simulink model "AA_Assemblage"  (R2020b)
settings: Solver=FixedStepAuto  StartTime=0.0  StopTime=inf  FixedStep=0.001  RelTol=1e-3
values from neighbouring files (symbols this model uses):
  smiData =     [A_robot_move.mat]
undefined symbols (not defined in the file or in its folder): Levenberg, Marquardt, W, X, Y, Z
libraries: sm_lib x1154, nesl_utility x40, robotlib x9, robotmaniplib x4, robotcorelib x2, simulink x1
(part 5 of 19)

== system AA_Assemblage/Robot_consigne/Poignet_1/SKF_7202_1_RIGID ==
  ReferenceFrame : sm_lib/Frames and Transforms/Reference Frame
  Solid : sm_lib/Body Elements/File Solid  ExtGeomFileName=SKF 7202.step  UnitType=FromFile  ExtGeomFileUnits=m  StepReaderType=HEX  ExportConvexHullGeometry=off  InertiaType=Custom  Mass=smiData.Solid(18).mass  MassUnits=kg  CenterOfMass=smiData.Solid(18).CoM  CenterOfMassUnits=mm  MomentsOfInertia=smiData.Solid(18).MoI  MomentsOfInertiaUnits=kg*mm^2  ProductsOfInertia=smiData.Solid(18).PoI  ProductsOfInertiaUnits=kg*mm^2  BasedOnType=DensityFromFile  Density=1000  DensityUnits=kg/m^3  DoExposeReferenceFrame=on  SerializedFrames=<Frames/>  GraphicType=FromGeometry  MarkerShape=Sphere  MarkerSize=10  GraphicVisPropType=SimpleVisualProperties  GraphicDiffuseColor=smiData.Solid(18).color  GraphicSpecularColor=[0.5 0.5 0.5 1.0]  GraphicAmbientColor=[0.15 0.15 0.15 1.0]  GraphicEmissiveColor=[0.0 0.0 0.0 1.0]  GraphicShininess=75  GraphicOpacity=smiData.Solid(18).opacity
  Transform : sm_lib/Frames and Transforms/Rigid Transform  TranslationMethod=Cartesian  TranslationStandardOffset=0  TranslationLengthUnit=mm  TranslationStandardAxis=+Z  TranslationCartesianOffset=smiData.RigidTransform(68).translation  TranslationROffset=0  TranslationROffsetUnits=m  TranslationZOffset=0  TranslationZOffsetUnits=m  TranslationThetaOffset=0  TranslationThetaOffsetUnits=deg  RotationMethod=ArbitraryAxis  RotationAngleUnits=rad  RotationStandardAxis=+Z  RotationAngle=smiData.RigidTransform(68).angle  RotationArbitraryAxis=smiData.RigidTransform(68).axis  FollAlignAxisA=+X  BaseAlignAxisA=+Y  FollAlignAxisB=+Y  BaseAlignAxisB=+Z  RotationSequenceAxes=FollowerAxes  RotationSequence=XYX  RotationSequenceAngles=[0 0 0]  RotationSequenceAnglesUnits=deg  RotationMatrix=[1 0 0; 0 1 0; 0 0 1]
  F : PMIOPort  Side=Left
  connections:
  ReferenceFrame/RConn1 -- Solid/RConn1 -- Transform/LConn1
  Transform/RConn1 -- F/RConn1

== system AA_Assemblage/Robot_consigne/Poignet_1/SKF_7202_2_RIGID ==
  ReferenceFrame : sm_lib/Frames and Transforms/Reference Frame
  Solid : sm_lib/Body Elements/File Solid  ExtGeomFileName=SKF 7202.step  UnitType=FromFile  ExtGeomFileUnits=m  StepReaderType=HEX  ExportConvexHullGeometry=off  InertiaType=Custom  Mass=smiData.Solid(18).mass  MassUnits=kg  CenterOfMass=smiData.Solid(18).CoM  CenterOfMassUnits=mm  MomentsOfInertia=smiData.Solid(18).MoI  MomentsOfInertiaUnits=kg*mm^2  ProductsOfInertia=smiData.Solid(18).PoI  ProductsOfInertiaUnits=kg*mm^2  BasedOnType=DensityFromFile  Density=1000  DensityUnits=kg/m^3  DoExposeReferenceFrame=on  SerializedFrames=<Frames/>  GraphicType=FromGeometry  MarkerShape=Sphere  MarkerSize=10  GraphicVisPropType=SimpleVisualProperties  GraphicDiffuseColor=smiData.Solid(18).color  GraphicSpecularColor=[0.5 0.5 0.5 1.0]  GraphicAmbientColor=[0.15 0.15 0.15 1.0]  GraphicEmissiveColor=[0.0 0.0 0.0 1.0]  GraphicShininess=75  GraphicOpacity=smiData.Solid(18).opacity
  Transform : sm_lib/Frames and Transforms/Rigid Transform  TranslationMethod=Cartesian  TranslationStandardOffset=0  TranslationLengthUnit=mm  TranslationStandardAxis=+Z  TranslationCartesianOffset=smiData.RigidTransform(78).translation  TranslationROffset=0  TranslationROffsetUnits=m  TranslationZOffset=0  TranslationZOffsetUnits=m  TranslationThetaOffset=0  TranslationThetaOffsetUnits=deg  RotationMethod=ArbitraryAxis  RotationAngleUnits=rad  RotationStandardAxis=+Z  RotationAngle=smiData.RigidTransform(78).angle  RotationArbitraryAxis=smiData.RigidTransform(78).axis  FollAlignAxisA=+X  BaseAlignAxisA=+Y  FollAlignAxisB=+Y  BaseAlignAxisB=+Z  RotationSequenceAxes=FollowerAxes  RotationSequence=XYX  RotationSequenceAngles=[0 0 0]  RotationSequenceAnglesUnits=deg  RotationMatrix=[1 0 0; 0 1 0; 0 0 1]
  Transform1 : sm_lib/Frames and Transforms/Rigid Transform  TranslationMethod=Cartesian  TranslationStandardOffset=0  TranslationLengthUnit=mm  TranslationStandardAxis=+Z  TranslationCartesianOffset=smiData.RigidTransform(97).translation  TranslationROffset=0  TranslationROffsetUnits=m  TranslationZOffset=0  TranslationZOffsetUnits=m  TranslationThetaOffset=0  TranslationThetaOffsetUnits=deg  RotationMethod=ArbitraryAxis  RotationAngleUnits=rad  RotationStandardAxis=+Z  RotationAngle=smiData.RigidTransform(97).angle  RotationArbitraryAxis=smiData.RigidTransform(97).axis  FollAlignAxisA=+X  BaseAlignAxisA=+Y  FollAlignAxisB=+Y  BaseAlignAxisB=+Z  RotationSequenceAxes=FollowerAxes  RotationSequence=XYX  RotationSequenceAngles=[0 0 0]  RotationSequenceAnglesUnits=deg  RotationMatrix=[1 0 0; 0 1 0; 0 0 1]
  F : PMIOPort  Side=Left
  F1 : PMIOPort  Port=2  Side=Left
  connections:
  ReferenceFrame/RConn1 -- Solid/RConn1 -- Transform/LConn1 -- Transform1/LConn1
  Transform/RConn1 -- F/RConn1
  Transform1/RConn1 -- F1/RConn1

== system AA_Assemblage/Robot_consigne/Poignet_1/Support_Rou_dente_coude_et_poignet_1_RIGID ==
  ReferenceFrame : sm_lib/Frames and Transforms/Reference Frame
  Solid : sm_lib/Body Elements/File Solid  ExtGeomFileName=Support Roué dentée coude et poignet.step  UnitType=FromFile  ExtGeomFileUnits=m  StepReaderType=HEX  ExportConvexHullGeometry=off  InertiaType=Custom  Mass=smiData.Solid(17).mass  MassUnits=kg  CenterOfMass=smiData.Solid(17).CoM  CenterOfMassUnits=mm  MomentsOfInertia=smiData.Solid(17).MoI  MomentsOfInertiaUnits=kg*mm^2  ProductsOfInertia=smiData.Solid(17).PoI  ProductsOfInertiaUnits=kg*mm^2  BasedOnType=DensityFromFile  Density=1000  DensityUnits=kg/m^3  DoExposeReferenceFrame=on  SerializedFrames=<Frames/>  GraphicType=FromGeometry  MarkerShape=Sphere  MarkerSize=10  GraphicVisPropType=SimpleVisualProperties  GraphicDiffuseColor=smiData.Solid(17).color  GraphicSpecularColor=[0.5 0.5 0.5 1.0]  GraphicAmbientColor=[0.15 0.15 0.15 1.0]  GraphicEmissiveColor=[0.0 0.0 0.0 1.0]  GraphicShininess=75  GraphicOpacity=smiData.Solid(17).opacity
  Transform : sm_lib/Frames and Transforms/Rigid Transform  TranslationMethod=Cartesian  TranslationStandardOffset=0  TranslationLengthUnit=mm  TranslationStandardAxis=+Z  TranslationCartesianOffset=smiData.RigidTransform(80).translation  TranslationROffset=0  TranslationROffsetUnits=m  TranslationZOffset=0  TranslationZOffsetUnits=m  TranslationThetaOffset=0  TranslationThetaOffsetUnits=deg  RotationMethod=ArbitraryAxis  RotationAngleUnits=rad  RotationStandardAxis=+Z  RotationAngle=smiData.RigidTransform(80).angle  RotationArbitraryAxis=smiData.RigidTransform(80).axis  FollAlignAxisA=+X  BaseAlignAxisA=+Y  FollAlignAxisB=+Y  BaseAlignAxisB=+Z  RotationSequenceAxes=FollowerAxes  RotationSequence=XYX  RotationSequenceAngles=[0 0 0]  RotationSequenceAnglesUnits=deg  RotationMatrix=[1 0 0; 0 1 0; 0 0 1]
  F : PMIOPort  Side=Left
  connections:
  ReferenceFrame/RConn1 -- Solid/RConn1 -- Transform/LConn1
  Transform/RConn1 -- F/RConn1

== system AA_Assemblage/Robot_consigne/Poignet_1/XL430_1_RIGID ==
  ReferenceFrame : sm_lib/Frames and Transforms/Reference Frame
  Solid : sm_lib/Body Elements/File Solid  ExtGeomFileName=XL430.step  UnitType=FromFile  ExtGeomFileUnits=m  StepReaderType=HEX  ExportConvexHullGeometry=off  InertiaType=Custom  Mass=smiData.Solid(22).mass  MassUnits=kg  CenterOfMass=smiData.Solid(22).CoM  CenterOfMassUnits=mm  MomentsOfInertia=smiData.Solid(22).MoI  MomentsOfInertiaUnits=kg*mm^2  ProductsOfInertia=smiData.Solid(22).PoI  ProductsOfInertiaUnits=kg*mm^2  BasedOnType=DensityFromFile  Density=1000  DensityUnits=kg/m^3  DoExposeReferenceFrame=on  SerializedFrames=<Frames/>  GraphicType=FromGeometry  MarkerShape=Sphere  MarkerSize=10  GraphicVisPropType=SimpleVisualProperties  GraphicDiffuseColor=smiData.Solid(22).color  GraphicSpecularColor=[0.5 0.5 0.5 1.0]  GraphicAmbientColor=[0.15 0.15 0.15 1.0]  GraphicEmissiveColor=[0.0 0.0 0.0 1.0]  GraphicShininess=75  GraphicOpacity=smiData.Solid(22).opacity
  Transform : sm_lib/Frames and Transforms/Rigid Transform  TranslationMethod=Cartesian  TranslationStandardOffset=0  TranslationLengthUnit=mm  TranslationStandardAxis=+Z  TranslationCartesianOffset=smiData.RigidTransform(76).translation  TranslationROffset=0  TranslationROffsetUnits=m  TranslationZOffset=0  TranslationZOffsetUnits=m  TranslationThetaOffset=0  TranslationThetaOffsetUnits=deg  RotationMethod=ArbitraryAxis  RotationAngleUnits=rad  RotationStandardAxis=+Z  RotationAngle=smiData.RigidTransform(76).angle  RotationArbitraryAxis=smiData.RigidTransform(76).axis  FollAlignAxisA=+X  BaseAlignAxisA=+Y  FollAlignAxisB=+Y  BaseAlignAxisB=+Z  RotationSequenceAxes=FollowerAxes  RotationSequence=XYX  RotationSequenceAngles=[0 0 0]  RotationSequenceAnglesUnits=deg  RotationMatrix=[1 0 0; 0 1 0; 0 0 1]
  Transform1 : sm_lib/Frames and Transforms/Rigid Transform  TranslationMethod=Cartesian  TranslationStandardOffset=0  TranslationLengthUnit=mm  TranslationStandardAxis=+Z  TranslationCartesianOffset=smiData.RigidTransform(79).translation  TranslationROffset=0  TranslationROffsetUnits=m  TranslationZOffset=0  TranslationZOffsetUnits=m  TranslationThetaOffset=0  TranslationThetaOffsetUnits=deg  RotationMethod=ArbitraryAxis  RotationAngleUnits=rad  RotationStandardAxis=+Z  RotationAngle=smiData.RigidTransform(79).angle  RotationArbitraryAxis=smiData.RigidTransform(79).axis  FollAlignAxisA=+X  BaseAlignAxisA=+Y  FollAlignAxisB=+Y  BaseAlignAxisB=+Z  RotationSequenceAxes=FollowerAxes  RotationSequence=XYX  RotationSequenceAngles=[0 0 0]  RotationSequenceAnglesUnits=deg  RotationMatrix=[1 0 0; 0 1 0; 0 0 1]
  F1 : PMIOPort  Side=Left
  F : PMIOPort  Port=2  Side=Left
  connections:
  ReferenceFrame/RConn1 -- Solid/RConn1 -- Transform/LConn1 -- Transform1/LConn1
  Transform/RConn1 -- F/RConn1
  Transform1/RConn1 -- F1/RConn1

== system AA_Assemblage/Subsystem1/Robot_verif/Base_1 ==
  Base_Complment_1_RIGID : Subsystem
  Couvercle_Base_1_RIGID : Subsystem
  Paroi_2_Base_1_RIGID : Subsystem
  Paroi_3_Base_1_RIGID : Subsystem
  Paroi_4_Base_1_RIGID : Subsystem
  Petite_Roue_dente_Bassin_1_RIGID : Subsystem
  ReferenceFrame : sm_lib/Frames and Transforms/Reference Frame
  ReferenceFrame1 : sm_lib/Frames and Transforms/Reference Frame
  SKF_7208_1_RIGID : Subsystem
  SKF_7208_2_RIGID : Subsystem
  Sol_Base_1_RIGID : Subsystem
  Support_Rou_dente_Base_1_RIGID : Subsystem
  Transform : sm_lib/Frames and Transforms/Rigid Transform  TranslationMethod=Cartesian  TranslationStandardOffset=0  TranslationLengthUnit=mm  TranslationStandardAxis=+Z  TranslationCartesianOffset=smiData.RigidTransform(103).translation  TranslationROffset=0  TranslationROffsetUnits=m  TranslationZOffset=0  TranslationZOffsetUnits=m  TranslationThetaOffset=0  TranslationThetaOffsetUnits=deg  RotationMethod=ArbitraryAxis  RotationAngleUnits=rad  RotationStandardAxis=+Z  RotationAngle=smiData.RigidTransform(103).angle  RotationArbitraryAxis=smiData.RigidTransform(103).axis  FollAlignAxisA=+X  BaseAlignAxisA=+Y  FollAlignAxisB=+Y  BaseAlignAxisB=+Z  RotationSequenceAxes=FollowerAxes  RotationSequence=XYX  RotationSequenceAngles=[0 0 0]  RotationSequenceAnglesUnits=deg  RotationMatrix=[1 0 0; 0 1 0; 0 0 1]
  Transform1 : sm_lib/Frames and Transforms/Rigid Transform  TranslationMethod=Cartesian  TranslationStandardOffset=0  TranslationLengthUnit=mm  TranslationStandardAxis=+Z  TranslationCartesianOffset=smiData.RigidTransform(106).translation  TranslationROffset=0  TranslationROffsetUnits=m  TranslationZOffset=0  TranslationZOffsetUnits=m  TranslationThetaOffset=0  TranslationThetaOffsetUnits=deg  RotationMethod=ArbitraryAxis  RotationAngleUnits=rad  RotationStandardAxis=+Z  RotationAngle=smiData.RigidTransform(106).angle  RotationArbitraryAxis=smiData.RigidTransform(106).axis  FollAlignAxisA=+X  BaseAlignAxisA=+Y  FollAlignAxisB=+Y  BaseAlignAxisB=+Z  RotationSequenceAxes=FollowerAxes  RotationSequence=XYX  RotationSequenceAngles=[0 0 0]  RotationSequenceAnglesUnits=deg  RotationMatrix=[1 0 0; 0 1 0; 0 0 1]
  XL430_1_RIGID : Subsystem
  F : PMIOPort  Side=Right
  F3 : PMIOPort  Port=2  Side=Left
  connections:
  Paroi_4_Base_1_RIGID/LConn1 -- Sol_Base_1_RIGID/LConn2 -- Paroi_2_Base_1_RIGID/LConn1 -- Paroi_3_Base_1_RIGID/LConn1
  Support_Rou_dente_Base_1_RIGID/LConn2 -- XL430_1_RIGID/LConn1
  ReferenceFrame/RConn1 -- Transform/LConn1
  Couvercle_Base_1_RIGID/LConn1 -- XL430_1_RIGID/LConn2
  Base_Complment_1_RIGID/LConn3 -- Sol_Base_1_RIGID/LConn1
  Petite_Roue_dente_Bassin_1_RIGID/LConn1 -- Support_Rou_dente_Base_1_RIGID/LConn1
  Base_Complment_1_RIGID/LConn1 -- Couvercle_Base_1_RIGID/LConn3
  Base_Complment_1_RIGID/LConn2 -- SKF_7208_1_RIGID/LConn2
  Base_Complment_1_RIGID/LConn4 -- SKF_7208_2_RIGID/LConn1
  SKF_7208_1_RIGID/LConn1 -- F/RConn1
  Couvercle_Base_1_RIGID/LConn2 -- Transform/RConn1
  F3/RConn1 -- Transform1/LConn1 -- ReferenceFrame1/RConn1
  Transform1/RConn1 -- Sol_Base_1_RIGID/LConn3

== system AA_Assemblage/Subsystem1/Robot_verif/Coude_1 ==
  Adaptateur_Arbre_01_1_RIGID : Subsystem
  Arbre_1_1_RIGID : Subsystem
  Bras_1_droite_1_RIGID : Subsystem
  Bras_1_gauche_1_RIGID : Subsystem
  Grande_Roue_dente_paule_1_RIGID : Subsystem
  Petite_Roue_dente_Coude_1_RIGID : Subsystem
  ReferenceFrame : sm_lib/Frames and Transforms/Reference Frame
  SKF_7202_1_RIGID : Subsystem
  SKF_7202_2_RIGID : Subsystem
  Support_Rou_dente_coude_et_poignet_1_RIGID : Subsystem
  XL430_1_RIGID : Subsystem
  F1 : PMIOPort  Side=Left
  F : PMIOPort  Port=2  Side=Right
  connections:
  Bras_1_droite_1_RIGID/LConn2 -- SKF_7202_1_RIGID/LConn2
  Bras_1_droite_1_RIGID/LConn1 -- XL430_1_RIGID/LConn2
  Adaptateur_Arbre_01_1_RIGID/LConn2 -- F1/RConn1
  Arbre_1_1_RIGID/LConn2 -- Bras_1_droite_1_RIGID/LConn3
  Support_Rou_dente_coude_et_poignet_1_RIGID/LConn2 -- XL430_1_RIGID/LConn1
  Adaptateur_Arbre_01_1_RIGID/LConn3 -- Grande_Roue_dente_paule_1_RIGID/LConn1
  Arbre_1_1_RIGID/LConn1 -- Bras_1_gauche_1_RIGID/LConn2
  Adaptateur_Arbre_01_1_RIGID/LConn1 -- Arbre_1_1_RIGID/LConn3
  Bras_1_gauche_1_RIGID/LConn1 -- SKF_7202_2_RIGID/LConn1
  Petite_Roue_dente_Coude_1_RIGID/LConn1 -- Support_Rou_dente_coude_et_poignet_1_RIGID/LConn1
  SKF_7202_1_RIGID/LConn1 -- F/RConn1

== system AA_Assemblage/Subsystem1/Robot_verif/Epaule_1 ==
  Bras_01_droite_3_RIGID : Subsystem
  Bras_01_gauche_4_RIGID : Subsystem
  Mt_1_RIGID : Subsystem
  Part_2_1_RIGID : Subsystem
  Petite_Roue_dente_paule_1_RIGID : Subsystem
  Plateau_complmentaire_du_mt_2_RIGID : Subsystem
  ReferenceFrame : sm_lib/Frames and Transforms/Reference Frame
  SKF_7202_1_RIGID : Subsystem
  SKF_7202_2_RIGID : Subsystem
  XL430_1_RIGID : Subsystem
  F1 : PMIOPort  Side=Left
  F : PMIOPort  Port=2  Side=Right
  connections:
  Petite_Roue_dente_paule_1_RIGID/LConn1 -- XL430_1_RIGID/LConn1
  Mt_1_RIGID/LConn5 -- Part_2_1_RIGID/LConn1
  Bras_01_gauche_4_RIGID/LConn3 -- Mt_1_RIGID/LConn2
  Mt_1_RIGID/LConn4 -- Plateau_complmentaire_du_mt_2_RIGID/LConn1
  Bras_01_droite_3_RIGID/LConn2 -- Mt_1_RIGID/LConn1
  Bras_01_gauche_4_RIGID/LConn1 -- XL430_1_RIGID/LConn2
  Bras_01_gauche_4_RIGID/LConn2 -- SKF_7202_2_RIGID/LConn1
  Bras_01_droite_3_RIGID/LConn1 -- SKF_7202_1_RIGID/LConn2
  SKF_7202_1_RIGID/LConn1 -- F/RConn1
  Mt_1_RIGID/LConn3 -- F1/RConn1

== system AA_Assemblage/Subsystem1/Robot_verif/Main_1 ==
  Arbre_Poignet_1_RIGID : Subsystem
  Main_assemble_1 : Subsystem
  Poignet_1_RIGID : Subsystem
  engrenage_sortie_1_RIGID : Subsystem
  F : PMIOPort  Side=Left
  F1 : PMIOPort  Port=2  Side=Right
  connections:
  Arbre_Poignet_1_RIGID/LConn3 -- engrenage_sortie_1_RIGID/LConn1
  Main_assemble_1/LConn1 -- Poignet_1_RIGID/LConn1
  Arbre_Poignet_1_RIGID/LConn1 -- Poignet_1_RIGID/LConn2
  Arbre_Poignet_1_RIGID/LConn2 -- F/RConn1
  F1/RConn1 -- Main_assemble_1/RConn1

== system AA_Assemblage/Subsystem1/Robot_verif/Poignet_1 ==
  Bras1_1_RIGID : Subsystem
  Grande_Roue_dente_Coude_1_RIGID : Subsystem
  Part_1_1_RIGID : Subsystem
  Part_2_1_RIGID : Subsystem
  ReferenceFrame : sm_lib/Frames and Transforms/Reference Frame
  SKF_7202_1_RIGID : Subsystem
  SKF_7202_2_RIGID : Subsystem
  Support_Rou_dente_coude_et_poignet_1_RIGID : Subsystem
  XL430_1_RIGID : Subsystem
  F : PMIOPort  Side=Left
  F1 : PMIOPort  Port=2  Side=Right
  connections:
  Bras1_1_RIGID/LConn3 -- SKF_7202_1_RIGID/LConn1
  Bras1_1_RIGID/LConn2 -- Part_1_1_RIGID/LConn3
  Part_1_1_RIGID/LConn4 -- Part_2_1_RIGID/LConn1
  Grande_Roue_dente_Coude_1_RIGID/LConn1 -- Part_1_1_RIGID/LConn1
  Bras1_1_RIGID/LConn1 -- XL430_1_RIGID/LConn2
  Part_2_1_RIGID/LConn2 -- SKF_7202_2_RIGID/LConn1
  Support_Rou_dente_coude_et_poignet_1_RIGID/LConn1 -- XL430_1_RIGID/LConn1
  Part_1_1_RIGID/LConn2 -- F/RConn1
  SKF_7202_2_RIGID/LConn2 -- F1/RConn1

== system AA_Assemblage/Subsystem2/Robot_verif/Base_1 ==
  Base_Complment_1_RIGID : Subsystem
  Couvercle_Base_1_RIGID : Subsystem
  Paroi_2_Base_1_RIGID : Subsystem
  Paroi_3_Base_1_RIGID : Subsystem
  Paroi_4_Base_1_RIGID : Subsystem
  Petite_Roue_dente_Bassin_1_RIGID : Subsystem
  ReferenceFrame : sm_lib/Frames and Transforms/Reference Frame
  ReferenceFrame1 : sm_lib/Frames and Transforms/Reference Frame
  SKF_7208_1_RIGID : Subsystem
  SKF_7208_2_RIGID : Subsystem
  Sol_Base_1_RIGID : Subsystem
  Support_Rou_dente_Base_1_RIGID : Subsystem
  Transform : sm_lib/Frames and Transforms/Rigid Transform  TranslationMethod=Cartesian  TranslationStandardOffset=0  TranslationLengthUnit=mm  TranslationStandardAxis=+Z  TranslationCartesianOffset=smiData.RigidTransform(103).translation  TranslationROffset=0  TranslationROffsetUnits=m  TranslationZOffset=0  TranslationZOffsetUnits=m  TranslationThetaOffset=0  TranslationThetaOffsetUnits=deg  RotationMethod=ArbitraryAxis  RotationAngleUnits=rad  RotationStandardAxis=+Z  RotationAngle=smiData.RigidTransform(103).angle  RotationArbitraryAxis=smiData.RigidTransform(103).axis  FollAlignAxisA=+X  BaseAlignAxisA=+Y  FollAlignAxisB=+Y  BaseAlignAxisB=+Z  RotationSequenceAxes=FollowerAxes  RotationSequence=XYX  RotationSequenceAngles=[0 0 0]  RotationSequenceAnglesUnits=deg  RotationMatrix=[1 0 0; 0 1 0; 0 0 1]
  Transform1 : sm_lib/Frames and Transforms/Rigid Transform  TranslationMethod=Cartesian  TranslationStandardOffset=0  TranslationLengthUnit=mm  TranslationStandardAxis=+Z  TranslationCartesianOffset=smiData.RigidTransform(106).translation  TranslationROffset=0  TranslationROffsetUnits=m  TranslationZOffset=0  TranslationZOffsetUnits=m  TranslationThetaOffset=0  TranslationThetaOffsetUnits=deg  RotationMethod=ArbitraryAxis  RotationAngleUnits=rad  RotationStandardAxis=+Z  RotationAngle=smiData.RigidTransform(106).angle  RotationArbitraryAxis=smiData.RigidTransform(106).axis  FollAlignAxisA=+X  BaseAlignAxisA=+Y  FollAlignAxisB=+Y  BaseAlignAxisB=+Z  RotationSequenceAxes=FollowerAxes  RotationSequence=XYX  RotationSequenceAngles=[0 0 0]  RotationSequenceAnglesUnits=deg  RotationMatrix=[1 0 0; 0 1 0; 0 0 1]
  XL430_1_RIGID : Subsystem
  F : PMIOPort  Side=Right
  F3 : PMIOPort  Port=2  Side=Left
  connections:
  Paroi_3_Base_1_RIGID/LConn1 -- Paroi_4_Base_1_RIGID/LConn1 -- Sol_Base_1_RIGID/LConn2 -- Paroi_2_Base_1_RIGID/LConn1
  Support_Rou_dente_Base_1_RIGID/LConn2 -- XL430_1_RIGID/LConn1
  ReferenceFrame/RConn1 -- Transform/LConn1
  Couvercle_Base_1_RIGID/LConn1 -- XL430_1_RIGID/LConn2
  Base_Complment_1_RIGID/LConn3 -- Sol_Base_1_RIGID/LConn1
  Petite_Roue_dente_Bassin_1_RIGID/LConn1 -- Support_Rou_dente_Base_1_RIGID/LConn1
  Base_Complment_1_RIGID/LConn1 -- Couvercle_Base_1_RIGID/LConn3
  Base_Complment_1_RIGID/LConn2 -- SKF_7208_1_RIGID/LConn2
  Base_Complment_1_RIGID/LConn4 -- SKF_7208_2_RIGID/LConn1
  SKF_7208_1_RIGID/LConn1 -- F/RConn1
  Couvercle_Base_1_RIGID/LConn2 -- Transform/RConn1
  Transform1/LConn1 -- ReferenceFrame1/RConn1 -- F3/RConn1
  Transform1/RConn1 -- Sol_Base_1_RIGID/LConn3

== system AA_Assemblage/Subsystem2/Robot_verif/Coude_1 ==
  Adaptateur_Arbre_01_1_RIGID : Subsystem
  Arbre_1_1_RIGID : Subsystem
  Bras_1_droite_1_RIGID : Subsystem
  Bras_1_gauche_1_RIGID : Subsystem
  Grande_Roue_dente_paule_1_RIGID : Subsystem
  Petite_Roue_dente_Coude_1_RIGID : Subsystem
  ReferenceFrame : sm_lib/Frames and Transforms/Reference Frame
  SKF_7202_1_RIGID : Subsystem
  SKF_7202_2_RIGID : Subsystem
  Support_Rou_dente_coude_et_poignet_1_RIGID : Subsystem
  XL430_1_RIGID : Subsystem
  F1 : PMIOPort  Side=Left
  F : PMIOPort  Port=2  Side=Right
  connections:
  Bras_1_droite_1_RIGID/LConn2 -- SKF_7202_1_RIGID/LConn2
  Bras_1_droite_1_RIGID/LConn1 -- XL430_1_RIGID/LConn2
  Adaptateur_Arbre_01_1_RIGID/LConn2 -- F1/RConn1
  Arbre_1_1_RIGID/LConn2 -- Bras_1_droite_1_RIGID/LConn3
  Support_Rou_dente_coude_et_poignet_1_RIGID/LConn2 -- XL430_1_RIGID/LConn1
  Adaptateur_Arbre_01_1_RIGID/LConn3 -- Grande_Roue_dente_paule_1_RIGID/LConn1
  Arbre_1_1_RIGID/LConn1 -- Bras_1_gauche_1_RIGID/LConn2
  Adaptateur_Arbre_01_1_RIGID/LConn1 -- Arbre_1_1_RIGID/LConn3
  Bras_1_gauche_1_RIGID/LConn1 -- SKF_7202_2_RIGID/LConn1
  Petite_Roue_dente_Coude_1_RIGID/LConn1 -- Support_Rou_dente_coude_et_poignet_1_RIGID/LConn1
  SKF_7202_1_RIGID/LConn1 -- F/RConn1

== system AA_Assemblage/Subsystem2/Robot_verif/Epaule_1 ==
  Bras_01_droite_3_RIGID : Subsystem
  Bras_01_gauche_4_RIGID : Subsystem
  Mt_1_RIGID : Subsystem
  Part_2_1_RIGID : Subsystem
  Petite_Roue_dente_paule_1_RIGID : Subsystem
  Plateau_complmentaire_du_mt_2_RIGID : Subsystem
  ReferenceFrame : sm_lib/Frames and Transforms/Reference Frame
  SKF_7202_1_RIGID : Subsystem
  SKF_7202_2_RIGID : Subsystem
  XL430_1_RIGID : Subsystem
  F1 : PMIOPort  Side=Left
  F : PMIOPort  Port=2  Side=Right
  connections:
  Petite_Roue_dente_paule_1_RIGID/LConn1 -- XL430_1_RIGID/LConn1
  Mt_1_RIGID/LConn5 -- Part_2_1_RIGID/LConn1
  Bras_01_gauche_4_RIGID/LConn3 -- Mt_1_RIGID/LConn2
  Mt_1_RIGID/LConn4 -- Plateau_complmentaire_du_mt_2_RIGID/LConn1
  Bras_01_droite_3_RIGID/LConn2 -- Mt_1_RIGID/LConn1
  Bras_01_gauche_4_RIGID/LConn1 -- XL430_1_RIGID/LConn2
  Bras_01_gauche_4_RIGID/LConn2 -- SKF_7202_2_RIGID/LConn1
  Bras_01_droite_3_RIGID/LConn1 -- SKF_7202_1_RIGID/LConn2
  SKF_7202_1_RIGID/LConn1 -- F/RConn1
  Mt_1_RIGID/LConn3 -- F1/RConn1

== system AA_Assemblage/Subsystem2/Robot_verif/Main_1 ==
  Arbre_Poignet_1_RIGID : Subsystem
  Main_assemble_1 : Subsystem
  Poignet_1_RIGID : Subsystem
  engrenage_sortie_1_RIGID : Subsystem
  F : PMIOPort  Side=Left
  F1 : PMIOPort  Port=2  Side=Right
  connections:
  Arbre_Poignet_1_RIGID/LConn3 -- engrenage_sortie_1_RIGID/LConn1
  Main_assemble_1/LConn1 -- Poignet_1_RIGID/LConn1
  Arbre_Poignet_1_RIGID/LConn1 -- Poignet_1_RIGID/LConn2
  Arbre_Poignet_1_RIGID/LConn2 -- F/RConn1
  F1/RConn1 -- Main_assemble_1/RConn1

== system AA_Assemblage/Subsystem2/Robot_verif/Poignet_1 ==
  Bras1_1_RIGID : Subsystem
  Grande_Roue_dente_Coude_1_RIGID : Subsystem
  Part_1_1_RIGID : Subsystem
  Part_2_1_RIGID : Subsystem
  ReferenceFrame : sm_lib/Frames and Transforms/Reference Frame
  SKF_7202_1_RIGID : Subsystem
  SKF_7202_2_RIGID : Subsystem
  Support_Rou_dente_coude_et_poignet_1_RIGID : Subsystem
  XL430_1_RIGID : Subsystem
  F : PMIOPort  Side=Left
  F1 : PMIOPort  Port=2  Side=Right
  connections:
  Bras1_1_RIGID/LConn3 -- SKF_7202_1_RIGID/LConn1
  Bras1_1_RIGID/LConn2 -- Part_1_1_RIGID/LConn3
  Part_1_1_RIGID/LConn4 -- Part_2_1_RIGID/LConn1
  Grande_Roue_dente_Coude_1_RIGID/LConn1 -- Part_1_1_RIGID/LConn1
  Bras1_1_RIGID/LConn1 -- XL430_1_RIGID/LConn2
  Part_2_1_RIGID/LConn2 -- SKF_7202_2_RIGID/LConn1
  Support_Rou_dente_coude_et_poignet_1_RIGID/LConn1 -- XL430_1_RIGID/LConn1
  Part_1_1_RIGID/LConn2 -- F/RConn1
  SKF_7202_2_RIGID/LConn2 -- F1/RConn1

== system AA_Assemblage/Subsystem3/Robot_verif/Base_1 ==
  Base_Complment_1_RIGID : Subsystem
  Couvercle_Base_1_RIGID : Subsystem
  Paroi_2_Base_1_RIGID : Subsystem
  Paroi_3_Base_1_RIGID : Subsystem
  Paroi_4_Base_1_RIGID : Subsystem
  Petite_Roue_dente_Bassin_1_RIGID : Subsystem
  ReferenceFrame : sm_lib/Frames and Transforms/Reference Frame
  ReferenceFrame1 : sm_lib/Frames and Transforms/Reference Frame
  SKF_7208_1_RIGID : Subsystem
  SKF_7208_2_RIGID : Subsystem
  Sol_Base_1_RIGID : Subsystem
  Support_Rou_dente_Base_1_RIGID : Subsystem
  Transform : sm_lib/Frames and Transforms/Rigid Transform  TranslationMethod=Cartesian  TranslationStandardOffset=0  TranslationLengthUnit=mm  TranslationStandardAxis=+Z  TranslationCartesianOffset=smiData.RigidTransform(103).translation  TranslationROffset=0  TranslationROffsetUnits=m  TranslationZOffset=0  TranslationZOffsetUnits=m  TranslationThetaOffset=0  TranslationThetaOffsetUnits=deg  RotationMethod=ArbitraryAxis  RotationAngleUnits=rad  RotationStandardAxis=+Z  RotationAngle=smiData.RigidTransform(103).angle  RotationArbitraryAxis=smiData.RigidTransform(103).axis  FollAlignAxisA=+X  BaseAlignAxisA=+Y  FollAlignAxisB=+Y  BaseAlignAxisB=+Z  RotationSequenceAxes=FollowerAxes  RotationSequence=XYX  RotationSequenceAngles=[0 0 0]  RotationSequenceAnglesUnits=deg  RotationMatrix=[1 0 0; 0 1 0; 0 0 1]
  Transform1 : sm_lib/Frames and Transforms/Rigid Transform  TranslationMethod=Cartesian  TranslationStandardOffset=0  TranslationLengthUnit=mm  TranslationStandardAxis=+Z  TranslationCartesianOffset=smiData.RigidTransform(106).translation  TranslationROffset=0  TranslationROffsetUnits=m  TranslationZOffset=0  TranslationZOffsetUnits=m  TranslationThetaOffset=0  TranslationThetaOffsetUnits=deg  RotationMethod=ArbitraryAxis  RotationAngleUnits=rad  RotationStandardAxis=+Z  RotationAngle=smiData.RigidTransform(106).angle  RotationArbitraryAxis=smiData.RigidTransform(106).axis  FollAlignAxisA=+X  BaseAlignAxisA=+Y  FollAlignAxisB=+Y  BaseAlignAxisB=+Z  RotationSequenceAxes=FollowerAxes  RotationSequence=XYX  RotationSequenceAngles=[0 0 0]  RotationSequenceAnglesUnits=deg  RotationMatrix=[1 0 0; 0 1 0; 0 0 1]
  XL430_1_RIGID : Subsystem
  F : PMIOPort  Side=Right
  F3 : PMIOPort  Port=2  Side=Left
  connections:
  Paroi_4_Base_1_RIGID/LConn1 -- Sol_Base_1_RIGID/LConn2 -- Paroi_2_Base_1_RIGID/LConn1 -- Paroi_3_Base_1_RIGID/LConn1
  Support_Rou_dente_Base_1_RIGID/LConn2 -- XL430_1_RIGID/LConn1
  ReferenceFrame/RConn1 -- Transform/LConn1
  Couvercle_Base_1_RIGID/LConn1 -- XL430_1_RIGID/LConn2
  Base_Complment_1_RIGID/LConn3 -- Sol_Base_1_RIGID/LConn1
  Petite_Roue_dente_Bassin_1_RIGID/LConn1 -- Support_Rou_dente_Base_1_RIGID/LConn1
  Base_Complment_1_RIGID/LConn1 -- Couvercle_Base_1_RIGID/LConn3
  Base_Complment_1_RIGID/LConn2 -- SKF_7208_1_RIGID/LConn2
  Base_Complment_1_RIGID/LConn4 -- SKF_7208_2_RIGID/LConn1
  SKF_7208_1_RIGID/LConn1 -- F/RConn1
  Couvercle_Base_1_RIGID/LConn2 -- Transform/RConn1
  F3/RConn1 -- Transform1/LConn1 -- ReferenceFrame1/RConn1
  Transform1/RConn1 -- Sol_Base_1_RIGID/LConn3

== system AA_Assemblage/Subsystem3/Robot_verif/Coude_1 ==
  Adaptateur_Arbre_01_1_RIGID : Subsystem
  Arbre_1_1_RIGID : Subsystem
  Bras_1_droite_1_RIGID : Subsystem
  Bras_1_gauche_1_RIGID : Subsystem
  Grande_Roue_dente_paule_1_RIGID : Subsystem
  Petite_Roue_dente_Coude_1_RIGID : Subsystem
  ReferenceFrame : sm_lib/Frames and Transforms/Reference Frame
  SKF_7202_1_RIGID : Subsystem
  SKF_7202_2_RIGID : Subsystem
  Support_Rou_dente_coude_et_poignet_1_RIGID : Subsystem
  XL430_1_RIGID : Subsystem
  F1 : PMIOPort  Side=Left
  F : PMIOPort  Port=2  Side=Right
  connections:
  Bras_1_droite_1_RIGID/LConn2 -- SKF_7202_1_RIGID/LConn2
  Bras_1_droite_1_RIGID/LConn1 -- XL430_1_RIGID/LConn2
  Adaptateur_Arbre_01_1_RIGID/LConn2 -- F1/RConn1
  Arbre_1_1_RIGID/LConn2 -- Bras_1_droite_1_RIGID/LConn3
  Support_Rou_dente_coude_et_poignet_1_RIGID/LConn2 -- XL430_1_RIGID/LConn1
  Adaptateur_Arbre_01_1_RIGID/LConn3 -- Grande_Roue_dente_paule_1_RIGID/LConn1
  Arbre_1_1_RIGID/LConn1 -- Bras_1_gauche_1_RIGID/LConn2
  Adaptateur_Arbre_01_1_RIGID/LConn1 -- Arbre_1_1_RIGID/LConn3
  Bras_1_gauche_1_RIGID/LConn1 -- SKF_7202_2_RIGID/LConn1
  Petite_Roue_dente_Coude_1_RIGID/LConn1 -- Support_Rou_dente_coude_et_poignet_1_RIGID/LConn1
  SKF_7202_1_RIGID/LConn1 -- F/RConn1

== system AA_Assemblage/Subsystem3/Robot_verif/Epaule_1 ==
  Bras_01_droite_3_RIGID : Subsystem
  Bras_01_gauche_4_RIGID : Subsystem
  Mt_1_RIGID : Subsystem
  Part_2_1_RIGID : Subsystem
  Petite_Roue_dente_paule_1_RIGID : Subsystem
  Plateau_complmentaire_du_mt_2_RIGID : Subsystem
  ReferenceFrame : sm_lib/Frames and Transforms/Reference Frame
  SKF_7202_1_RIGID : Subsystem
  SKF_7202_2_RIGID : Subsystem
  XL430_1_RIGID : Subsystem
  F1 : PMIOPort  Side=Left
  F : PMIOPort  Port=2  Side=Right
  connections:
  Petite_Roue_dente_paule_1_RIGID/LConn1 -- XL430_1_RIGID/LConn1
  Mt_1_RIGID/LConn5 -- Part_2_1_RIGID/LConn1
  Bras_01_gauche_4_RIGID/LConn3 -- Mt_1_RIGID/LConn2
  Mt_1_RIGID/LConn4 -- Plateau_complmentaire_du_mt_2_RIGID/LConn1
  Bras_01_droite_3_RIGID/LConn2 -- Mt_1_RIGID/LConn1
  Bras_01_gauche_4_RIGID/LConn1 -- XL430_1_RIGID/LConn2
  Bras_01_gauche_4_RIGID/LConn2 -- SKF_7202_2_RIGID/LConn1
  Bras_01_droite_3_RIGID/LConn1 -- SKF_7202_1_RIGID/LConn2
  SKF_7202_1_RIGID/LConn1 -- F/RConn1
  Mt_1_RIGID/LConn3 -- F1/RConn1

== system AA_Assemblage/Subsystem3/Robot_verif/Main_1 ==
  Arbre_Poignet_1_RIGID : Subsystem
  Main_assemble_1 : Subsystem
  Poignet_1_RIGID : Subsystem
  engrenage_sortie_1_RIGID : Subsystem
  F : PMIOPort  Side=Left
  F1 : PMIOPort  Port=2  Side=Right
  F2 : PMIOPort  Port=3  Side=Right
  connections:
  Arbre_Poignet_1_RIGID/LConn3 -- engrenage_sortie_1_RIGID/LConn1
  Main_assemble_1/LConn1 -- Poignet_1_RIGID/LConn1
  Arbre_Poignet_1_RIGID/LConn1 -- Poignet_1_RIGID/LConn2
  Arbre_Poignet_1_RIGID/LConn2 -- F/RConn1
  F1/RConn1 -- Main_assemble_1/RConn1
  F2/RConn1 -- Main_assemble_1/RConn2

== system AA_Assemblage/Subsystem3/Robot_verif/Poignet_1 ==
  Bras1_1_RIGID : Subsystem
  Grande_Roue_dente_Coude_1_RIGID : Subsystem
  Part_1_1_RIGID : Subsystem
  Part_2_1_RIGID : Subsystem
  ReferenceFrame : sm_lib/Frames and Transforms/Reference Frame
  SKF_7202_1_RIGID : Subsystem
  SKF_7202_2_RIGID : Subsystem
  Support_Rou_dente_coude_et_poignet_1_RIGID : Subsystem
  XL430_1_RIGID : Subsystem
  F : PMIOPort  Side=Left
  F1 : PMIOPort  Port=2  Side=Right
  connections:
  Bras1_1_RIGID/LConn3 -- SKF_7202_1_RIGID/LConn1
  Bras1_1_RIGID/LConn2 -- Part_1_1_RIGID/LConn3
  Part_1_1_RIGID/LConn4 -- Part_2_1_RIGID/LConn1
  Grande_Roue_dente_Coude_1_RIGID/LConn1 -- Part_1_1_RIGID/LConn1
  Bras1_1_RIGID/LConn1 -- XL430_1_RIGID/LConn2
  Part_2_1_RIGID/LConn2 -- SKF_7202_2_RIGID/LConn1
  Support_Rou_dente_coude_et_poignet_1_RIGID/LConn1 -- XL430_1_RIGID/LConn1
  Part_1_1_RIGID/LConn2 -- F/RConn1
  SKF_7202_2_RIGID/LConn2 -- F1/RConn1

== system AA_Assemblage/bassin/epaule/coude ==
  In1 : Inport
  Add : Sum
  Constant : Constant  Value=-90
  For Iterator : ForIterator  ResetStates=reset
  Gain : Gain  Gain=20
  Mux : Mux  Inputs=2
  poignet : Subsystem  TreatAsAtomicUnit=on
  wires:
  Add/1 -> Mux/2
  Mux/1 -> poignet/1(In1)
  In1/1 -> Mux/1
  Constant/1 -> Add/2
  For Iterator/1 -> Gain/1
  Gain/1 -> Add/1

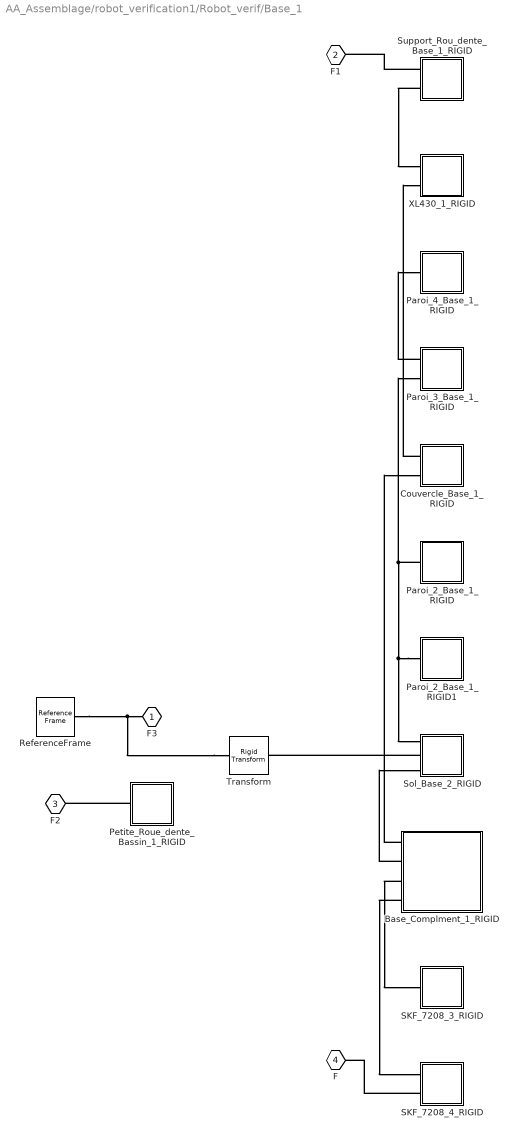
== system AA_Assemblage/robot_verification1/Robot_verif/Base_1 ==
  Base_Complment_1_RIGID : Subsystem
  Couvercle_Base_1_RIGID : Subsystem
  Paroi_2_Base_1_RIGID : Subsystem
  Paroi_2_Base_1_RIGID1 : Subsystem
  Paroi_3_Base_1_RIGID : Subsystem
  Paroi_4_Base_1_RIGID : Subsystem
  Petite_Roue_dente_Bassin_1_RIGID : Subsystem
  ReferenceFrame : sm_lib/Frames and Transforms/Reference Frame
  SKF_7208_3_RIGID : Subsystem
  SKF_7208_4_RIGID : Subsystem
  Sol_Base_2_RIGID : Subsystem
  Support_Rou_dente_Base_1_RIGID : Subsystem
  Transform : sm_lib/Frames and Transforms/Rigid Transform  TranslationMethod=Cartesian  TranslationStandardOffset=0  TranslationLengthUnit=mm  TranslationStandardAxis=+Z  TranslationCartesianOffset=smiData.RigidTransform(97).translation  TranslationROffset=0  TranslationROffsetUnits=m  TranslationZOffset=0  TranslationZOffsetUnits=m  TranslationThetaOffset=0  TranslationThetaOffsetUnits=deg  RotationMethod=ArbitraryAxis  RotationAngleUnits=rad  RotationStandardAxis=+Z  RotationAngle=smiData.RigidTransform(97).angle  RotationArbitraryAxis=smiData.RigidTransform(97).axis  FollAlignAxisA=+X  BaseAlignAxisA=+Y  FollAlignAxisB=+Y  BaseAlignAxisB=+Z  RotationSequenceAxes=FollowerAxes  RotationSequence=XYX  RotationSequenceAngles=[0 0 0]  RotationSequenceAnglesUnits=deg  RotationMatrix=[1 0 0; 0 1 0; 0 0 1]
  XL430_1_RIGID : Subsystem
  F3 : PMIOPort  Side=Left
  F1 : PMIOPort  Port=2  Side=Left
  F2 : PMIOPort  Port=3  Side=Left
  F : PMIOPort  Port=4  Side=Right
  connections:
  Paroi_2_Base_1_RIGID1/LConn1 -- Paroi_2_Base_1_RIGID/LConn1 -- Paroi_3_Base_1_RIGID/LConn2 -- Sol_Base_2_RIGID/LConn1
  Paroi_3_Base_1_RIGID/LConn1 -- Paroi_4_Base_1_RIGID/LConn1
  Petite_Roue_dente_Bassin_1_RIGID/LConn1 -- F2/RConn1
  Sol_Base_2_RIGID/LConn2 -- Transform/RConn1
  Transform/LConn1 -- ReferenceFrame/RConn1 -- F3/RConn1
  Support_Rou_dente_Base_1_RIGID/LConn2 -- XL430_1_RIGID/LConn1
  Base_Complment_1_RIGID/LConn4 -- SKF_7208_4_RIGID/LConn1
  Base_Complment_1_RIGID/LConn3 -- SKF_7208_3_RIGID/LConn1
  Base_Complment_1_RIGID/LConn2 -- Sol_Base_2_RIGID/LConn3
  Couvercle_Base_1_RIGID/LConn1 -- XL430_1_RIGID/LConn2
  Base_Complment_1_RIGID/LConn1 -- Couvercle_Base_1_RIGID/LConn2
  SKF_7208_4_RIGID/LConn2 -- F/RConn1
  Support_Rou_dente_Base_1_RIGID/LConn1 -- F1/RConn1

== system AA_Assemblage/robot_verification1/Robot_verif/Coude_1 ==
  Adaptateur_Arbre_01_1_RIGID : Subsystem
  Arbre_1_1_RIGID : Subsystem
  Bras_1_droite_1_RIGID : Subsystem
  Bras_1_gauche_1_RIGID : Subsystem
  Grande_Roue_dente_paule_1_RIGID : Subsystem
  ReferenceFrame : sm_lib/Frames and Transforms/Reference Frame
  SKF_7202_1_RIGID : Subsystem
  SKF_7202_2_RIGID : Subsystem
  XL430_1_RIGID : Subsystem
  F1 : PMIOPort  Side=Left
  F : PMIOPort  Port=2  Side=Right
  connections:
  Bras_1_droite_1_RIGID/LConn3 -- SKF_7202_1_RIGID/LConn1
  Bras_1_droite_1_RIGID/LConn2 -- XL430_1_RIGID/LConn1
  Arbre_1_1_RIGID/LConn4 -- Bras_1_droite_1_RIGID/LConn1
  Adaptateur_Arbre_01_1_RIGID/LConn2 -- Grande_Roue_dente_paule_1_RIGID/LConn1
  Arbre_1_1_RIGID/LConn1 -- Bras_1_gauche_1_RIGID/LConn2
  Adaptateur_Arbre_01_1_RIGID/LConn1 -- Arbre_1_1_RIGID/LConn3
  Bras_1_gauche_1_RIGID/LConn1 -- SKF_7202_2_RIGID/LConn2
  SKF_7202_2_RIGID/LConn1 -- F/RConn1
  Arbre_1_1_RIGID/LConn2 -- F1/RConn1

== system AA_Assemblage/robot_verification1/Robot_verif/Epaule_1 ==
  Bras_01_droite_3_RIGID : Subsystem
  Bras_01_gauche_4_RIGID : Subsystem
  Grande_Roue_dente_Bassin_1_RIGID : Subsystem
  Mt_1_RIGID : Subsystem
  Petite_Roue_dente_paule_1_RIGID : Subsystem
  Plateau_complmentaire_du_mt_2_RIGID : Subsystem
  ReferenceFrame : sm_lib/Frames and Transforms/Reference Frame
  SKF_7202_1_RIGID : Subsystem
  SKF_7202_2_RIGID : Subsystem
  XL430_1_RIGID : Subsystem
  F : PMIOPort  Side=Left
  F1 : PMIOPort  Port=2  Side=Right
  connections:
  Petite_Roue_dente_paule_1_RIGID/LConn1 -- XL430_1_RIGID/LConn1
  Grande_Roue_dente_Bassin_1_RIGID/LConn1 -- Mt_1_RIGID/LConn4
  Bras_01_gauche_4_RIGID/LConn3 -- Mt_1_RIGID/LConn1
  Mt_1_RIGID/LConn2 -- Plateau_complmentaire_du_mt_2_RIGID/LConn1
  Bras_01_droite_3_RIGID/LConn1 -- Mt_1_RIGID/LConn5
  Bras_01_gauche_4_RIGID/LConn1 -- XL430_1_RIGID/LConn2
  Bras_01_gauche_4_RIGID/LConn2 -- SKF_7202_2_RIGID/LConn2
  Bras_01_droite_3_RIGID/LConn2 -- SKF_7202_1_RIGID/LConn1
  Mt_1_RIGID/LConn3 -- F/RConn1
  SKF_7202_2_RIGID/LConn1 -- F1/RConn1

== system AA_Assemblage/robot_verification1/Robot_verif/Main_1 ==
  Arbre_Poignet_1_RIGID : Subsystem
  Main_assemble_1 : Subsystem
  Poignet_1_RIGID : Subsystem
  ReferenceFrame : sm_lib/Frames and Transforms/Reference Frame
  engrenage_sortie_1_RIGID : Subsystem
  F : PMIOPort  Side=Left
  F1 : PMIOPort  Port=2  Side=Right
  connections:
  Arbre_Poignet_1_RIGID/LConn2 -- engrenage_sortie_1_RIGID/LConn1
  Main_assemble_1/LConn1 -- Poignet_1_RIGID/LConn2
  Arbre_Poignet_1_RIGID/LConn1 -- Poignet_1_RIGID/LConn3
  Poignet_1_RIGID/LConn1 -- F/RConn1
  F1/RConn1 -- Main_assemble_1/RConn1

== system AA_Assemblage/robot_verification1/Robot_verif/Poignet_1 ==
  Arbre_12_1_RIGID : Subsystem
  Bras1_1_RIGID : Subsystem
  Grande_Roue_dente_Coude_1_RIGID : Subsystem
  Part_2_1_RIGID : Subsystem
  ReferenceFrame : sm_lib/Frames and Transforms/Reference Frame
  SKF_7202_1_RIGID : Subsystem
  SKF_7202_2_RIGID : Subsystem
  XL430_1_RIGID : Subsystem
  F1 : PMIOPort  Side=Left
  F : PMIOPort  Port=2  Side=Right
  connections:
  Bras1_1_RIGID/LConn3 -- SKF_7202_1_RIGID/LConn1
  Arbre_12_1_RIGID/LConn4 -- Bras1_1_RIGID/LConn1
  Bras1_1_RIGID/LConn2 -- XL430_1_RIGID/LConn1
  Arbre_12_1_RIGID/LConn3 -- Part_2_1_RIGID/LConn1
  Part_2_1_RIGID/LConn2 -- SKF_7202_2_RIGID/LConn1
  Arbre_12_1_RIGID/LConn1 -- Grande_Roue_dente_Coude_1_RIGID/LConn1
  SKF_7202_1_RIGID/LConn2 -- F/RConn1
  Arbre_12_1_RIGID/LConn2 -- F1/RConn1

== system AA_Assemblage/Robot_consigne/Main_1/Main_assemble_1/AX_12W_1_RIGID ==
  ReferenceFrame : sm_lib/Frames and Transforms/Reference Frame
  Solid : sm_lib/Body Elements/File Solid  ExtGeomFileName=AX_12W.step  UnitType=FromFile  ExtGeomFileUnits=m  StepReaderType=HEX  ExportConvexHullGeometry=off  InertiaType=Custom  Mass=smiData.Solid(4).mass  MassUnits=kg  CenterOfMass=smiData.Solid(4).CoM  CenterOfMassUnits=mm  MomentsOfInertia=smiData.Solid(4).MoI  MomentsOfInertiaUnits=kg*mm^2  ProductsOfInertia=smiData.Solid(4).PoI  ProductsOfInertiaUnits=kg*mm^2  BasedOnType=DensityFromFile  Density=1000  DensityUnits=kg/m^3  DoExposeReferenceFrame=on  SerializedFrames=<Frames/>  GraphicType=FromGeometry  MarkerShape=Sphere  MarkerSize=10  GraphicVisPropType=SimpleVisualProperties  GraphicDiffuseColor=smiData.Solid(4).color  GraphicSpecularColor=[0.5 0.5 0.5 1.0]  GraphicAmbientColor=[0.15 0.15 0.15 1.0]  GraphicEmissiveColor=[0.0 0.0 0.0 1.0]  GraphicShininess=75  GraphicOpacity=smiData.Solid(4).opacity
  Transform : sm_lib/Frames and Transforms/Rigid Transform  TranslationMethod=Cartesian  TranslationStandardOffset=0  TranslationLengthUnit=mm  TranslationStandardAxis=+Z  TranslationCartesianOffset=smiData.RigidTransform(9).translation  TranslationROffset=0  TranslationROffsetUnits=m  TranslationZOffset=0  TranslationZOffsetUnits=m  TranslationThetaOffset=0  TranslationThetaOffsetUnits=deg  RotationMethod=ArbitraryAxis  RotationAngleUnits=rad  RotationStandardAxis=+Z  RotationAngle=smiData.RigidTransform(9).angle  RotationArbitraryAxis=smiData.RigidTransform(9).axis  FollAlignAxisA=+X  BaseAlignAxisA=+Y  FollAlignAxisB=+Y  BaseAlignAxisB=+Z  RotationSequenceAxes=FollowerAxes  RotationSequence=XYX  RotationSequenceAngles=[0 0 0]  RotationSequenceAnglesUnits=deg  RotationMatrix=[1 0 0; 0 1 0; 0 0 1]
  Transform1 : sm_lib/Frames and Transforms/Rigid Transform  TranslationMethod=Cartesian  TranslationStandardOffset=0  TranslationLengthUnit=mm  TranslationStandardAxis=+Z  TranslationCartesianOffset=smiData.RigidTransform(12).translation  TranslationROffset=0  TranslationROffsetUnits=m  TranslationZOffset=0  TranslationZOffsetUnits=m  TranslationThetaOffset=0  TranslationThetaOffsetUnits=deg  RotationMethod=ArbitraryAxis  RotationAngleUnits=rad  RotationStandardAxis=+Z  RotationAngle=smiData.RigidTransform(12).angle  RotationArbitraryAxis=smiData.RigidTransform(12).axis  FollAlignAxisA=+X  BaseAlignAxisA=+Y  FollAlignAxisB=+Y  BaseAlignAxisB=+Z  RotationSequenceAxes=FollowerAxes  RotationSequence=XYX  RotationSequenceAngles=[0 0 0]  RotationSequenceAnglesUnits=deg  RotationMatrix=[1 0 0; 0 1 0; 0 0 1]
  F1 : PMIOPort  Side=Left
  F : PMIOPort  Port=2  Side=Left
  connections:
  ReferenceFrame/RConn1 -- Solid/RConn1 -- Transform/LConn1 -- Transform1/LConn1
  Transform/RConn1 -- F/RConn1
  Transform1/RConn1 -- F1/RConn1

== system AA_Assemblage/Robot_consigne/Main_1/Main_assemble_1/Corps_1_RIGID ==
  ReferenceFrame : sm_lib/Frames and Transforms/Reference Frame
  Solid : sm_lib/Body Elements/File Solid  ExtGeomFileName=Corps.step  UnitType=FromFile  ExtGeomFileUnits=m  StepReaderType=HEX  ExportConvexHullGeometry=off  InertiaType=Custom  Mass=smiData.Solid(5).mass  MassUnits=kg  CenterOfMass=smiData.Solid(5).CoM  CenterOfMassUnits=mm  MomentsOfInertia=smiData.Solid(5).MoI  MomentsOfInertiaUnits=kg*mm^2  ProductsOfInertia=smiData.Solid(5).PoI  ProductsOfInertiaUnits=kg*mm^2  BasedOnType=DensityFromFile  Density=1000  DensityUnits=kg/m^3  DoExposeReferenceFrame=on  SerializedFrames=<Frames/>  GraphicType=FromGeometry  MarkerShape=Sphere  MarkerSize=10  GraphicVisPropType=SimpleVisualProperties  GraphicDiffuseColor=smiData.Solid(5).color  GraphicSpecularColor=[0.5 0.5 0.5 1.0]  GraphicAmbientColor=[0.15 0.15 0.15 1.0]  GraphicEmissiveColor=[0.0 0.0 0.0 1.0]  GraphicShininess=75  GraphicOpacity=smiData.Solid(5).opacity
  Transform : sm_lib/Frames and Transforms/Rigid Transform  TranslationMethod=Cartesian  TranslationStandardOffset=0  TranslationLengthUnit=mm  TranslationStandardAxis=+Z  TranslationCartesianOffset=smiData.RigidTransform(7).translation  TranslationROffset=0  TranslationROffsetUnits=m  TranslationZOffset=0  TranslationZOffsetUnits=m  TranslationThetaOffset=0  TranslationThetaOffsetUnits=deg  RotationMethod=ArbitraryAxis  RotationAngleUnits=rad  RotationStandardAxis=+Z  RotationAngle=smiData.RigidTransform(7).angle  RotationArbitraryAxis=smiData.RigidTransform(7).axis  FollAlignAxisA=+X  BaseAlignAxisA=+Y  FollAlignAxisB=+Y  BaseAlignAxisB=+Z  RotationSequenceAxes=FollowerAxes  RotationSequence=XYX  RotationSequenceAngles=[0 0 0]  RotationSequenceAnglesUnits=deg  RotationMatrix=[1 0 0; 0 1 0; 0 0 1]
  Transform1 : sm_lib/Frames and Transforms/Rigid Transform  TranslationMethod=Cartesian  TranslationStandardOffset=0  TranslationLengthUnit=mm  TranslationStandardAxis=+Z  TranslationCartesianOffset=smiData.RigidTransform(19).translation  TranslationROffset=0  TranslationROffsetUnits=m  TranslationZOffset=0  TranslationZOffsetUnits=m  TranslationThetaOffset=0  TranslationThetaOffsetUnits=deg  RotationMethod=ArbitraryAxis  RotationAngleUnits=rad  RotationStandardAxis=+Z  RotationAngle=smiData.RigidTransform(19).angle  RotationArbitraryAxis=smiData.RigidTransform(19).axis  FollAlignAxisA=+X  BaseAlignAxisA=+Y  FollAlignAxisB=+Y  BaseAlignAxisB=+Z  RotationSequenceAxes=FollowerAxes  RotationSequence=XYX  RotationSequenceAngles=[0 0 0]  RotationSequenceAnglesUnits=deg  RotationMatrix=[1 0 0; 0 1 0; 0 0 1]
  Transform2 : sm_lib/Frames and Transforms/Rigid Transform  TranslationMethod=Cartesian  TranslationStandardOffset=0  TranslationLengthUnit=mm  TranslationStandardAxis=+Z  TranslationCartesianOffset=smiData.RigidTransform(22).translation  TranslationROffset=0  TranslationROffsetUnits=m  TranslationZOffset=0  TranslationZOffsetUnits=m  TranslationThetaOffset=0  TranslationThetaOffsetUnits=deg  RotationMethod=ArbitraryAxis  RotationAngleUnits=rad  RotationStandardAxis=+Z  RotationAngle=smiData.RigidTransform(22).angle  RotationArbitraryAxis=smiData.RigidTransform(22).axis  FollAlignAxisA=+X  BaseAlignAxisA=+Y  FollAlignAxisB=+Y  BaseAlignAxisB=+Z  RotationSequenceAxes=FollowerAxes  RotationSequence=XYX  RotationSequenceAngles=[0 0 0]  RotationSequenceAnglesUnits=deg  RotationMatrix=[1 0 0; 0 1 0; 0 0 1]
  Transform3 : sm_lib/Frames and Transforms/Rigid Transform  TranslationMethod=Cartesian  TranslationStandardOffset=0  TranslationLengthUnit=mm  TranslationStandardAxis=+Z  TranslationCartesianOffset=smiData.RigidTransform(23).translation  TranslationROffset=0  TranslationROffsetUnits=m  TranslationZOffset=0  TranslationZOffsetUnits=m  TranslationThetaOffset=0  TranslationThetaOffsetUnits=deg  RotationMethod=ArbitraryAxis  RotationAngleUnits=rad  RotationStandardAxis=+Z  RotationAngle=smiData.RigidTransform(23).angle  RotationArbitraryAxis=smiData.RigidTransform(23).axis  FollAlignAxisA=+X  BaseAlignAxisA=+Y  FollAlignAxisB=+Y  BaseAlignAxisB=+Z  RotationSequenceAxes=FollowerAxes  RotationSequence=XYX  RotationSequenceAngles=[0 0 0]  RotationSequenceAnglesUnits=deg  RotationMatrix=[1 0 0; 0 1 0; 0 0 1]
  Transform4 : sm_lib/Frames and Transforms/Rigid Transform  TranslationMethod=Cartesian  TranslationStandardOffset=0  TranslationLengthUnit=mm  TranslationStandardAxis=+Z  TranslationCartesianOffset=smiData.RigidTransform(25).translation  TranslationROffset=0  TranslationROffsetUnits=m  TranslationZOffset=0  TranslationZOffsetUnits=m  TranslationThetaOffset=0  TranslationThetaOffsetUnits=deg  RotationMethod=ArbitraryAxis  RotationAngleUnits=rad  RotationStandardAxis=+Z  RotationAngle=smiData.RigidTransform(25).angle  RotationArbitraryAxis=smiData.RigidTransform(25).axis  FollAlignAxisA=+X  BaseAlignAxisA=+Y  FollAlignAxisB=+Y  BaseAlignAxisB=+Z  RotationSequenceAxes=FollowerAxes  RotationSequence=XYX  RotationSequenceAngles=[0 0 0]  RotationSequenceAnglesUnits=deg  RotationMatrix=[1 0 0; 0 1 0; 0 0 1]
  F3 : PMIOPort  Side=Left
  F2 : PMIOPort  Port=2  Side=Left
  F4 : PMIOPort  Port=3  Side=Left
  F1 : PMIOPort  Port=4  Side=Left
  F : PMIOPort  Port=5  Side=Left
  connections:
  ReferenceFrame/RConn1 -- Solid/RConn1 -- Transform/LConn1 -- Transform1/LConn1 -- Transform2/LConn1 -- Transform3/LConn1 -- Transform4/LConn1
  Transform/RConn1 -- F/RConn1
  Transform1/RConn1 -- F1/RConn1
  Transform2/RConn1 -- F2/RConn1
  Transform3/RConn1 -- F3/RConn1
  Transform4/RConn1 -- F4/RConn1

== system AA_Assemblage/Robot_consigne/Main_1/Main_assemble_1/Couvercle_1_RIGID ==
  ReferenceFrame : sm_lib/Frames and Transforms/Reference Frame
  Solid : sm_lib/Body Elements/File Solid  ExtGeomFileName=Couvercle.step  UnitType=FromFile  ExtGeomFileUnits=m  StepReaderType=HEX  ExportConvexHullGeometry=off  InertiaType=Custom  Mass=smiData.Solid(10).mass  MassUnits=kg  CenterOfMass=smiData.Solid(10).CoM  CenterOfMassUnits=mm  MomentsOfInertia=smiData.Solid(10).MoI  MomentsOfInertiaUnits=kg*mm^2  ProductsOfInertia=smiData.Solid(10).PoI  ProductsOfInertiaUnits=kg*mm^2  BasedOnType=DensityFromFile  Density=1000  DensityUnits=kg/m^3  DoExposeReferenceFrame=on  SerializedFrames=<Frames/>  GraphicType=FromGeometry  MarkerShape=Sphere  MarkerSize=10  GraphicVisPropType=SimpleVisualProperties  GraphicDiffuseColor=smiData.Solid(10).color  GraphicSpecularColor=[0.5 0.5 0.5 1.0]  GraphicAmbientColor=[0.15 0.15 0.15 1.0]  GraphicEmissiveColor=[0.0 0.0 0.0 1.0]  GraphicShininess=75  GraphicOpacity=smiData.Solid(10).opacity
  Transform : sm_lib/Frames and Transforms/Rigid Transform  TranslationMethod=Cartesian  TranslationStandardOffset=0  TranslationLengthUnit=mm  TranslationStandardAxis=+Z  TranslationCartesianOffset=smiData.RigidTransform(15).translation  TranslationROffset=0  TranslationROffsetUnits=m  TranslationZOffset=0  TranslationZOffsetUnits=m  TranslationThetaOffset=0  TranslationThetaOffsetUnits=deg  RotationMethod=ArbitraryAxis  RotationAngleUnits=rad  RotationStandardAxis=+Z  RotationAngle=smiData.RigidTransform(15).angle  RotationArbitraryAxis=smiData.RigidTransform(15).axis  FollAlignAxisA=+X  BaseAlignAxisA=+Y  FollAlignAxisB=+Y  BaseAlignAxisB=+Z  RotationSequenceAxes=FollowerAxes  RotationSequence=XYX  RotationSequenceAngles=[0 0 0]  RotationSequenceAnglesUnits=deg  RotationMatrix=[1 0 0; 0 1 0; 0 0 1]
  Transform1 : sm_lib/Frames and Transforms/Rigid Transform  TranslationMethod=Cartesian  TranslationStandardOffset=0  TranslationLengthUnit=mm  TranslationStandardAxis=+Z  TranslationCartesianOffset=smiData.RigidTransform(24).translation  TranslationROffset=0  TranslationROffsetUnits=m  TranslationZOffset=0  TranslationZOffsetUnits=m  TranslationThetaOffset=0  TranslationThetaOffsetUnits=deg  RotationMethod=ArbitraryAxis  RotationAngleUnits=rad  RotationStandardAxis=+Z  RotationAngle=smiData.RigidTransform(24).angle  RotationArbitraryAxis=smiData.RigidTransform(24).axis  FollAlignAxisA=+X  BaseAlignAxisA=+Y  FollAlignAxisB=+Y  BaseAlignAxisB=+Z  RotationSequenceAxes=FollowerAxes  RotationSequence=XYX  RotationSequenceAngles=[0 0 0]  RotationSequenceAnglesUnits=deg  RotationMatrix=[1 0 0; 0 1 0; 0 0 1]
  F : PMIOPort  Side=Left
  F1 : PMIOPort  Port=2  Side=Left
  connections:
  ReferenceFrame/RConn1 -- Solid/RConn1 -- Transform/LConn1 -- Transform1/LConn1
  Transform/RConn1 -- F/RConn1
  Transform1/RConn1 -- F1/RConn1
